simulink model "F1WingAeroDemo"  (R2025b)
settings: Solver=ode45  StartTime=0.0  StopTime=20  RelTol=1e-3
settings Model: Creator=logan78  LastModifiedBy=logan78

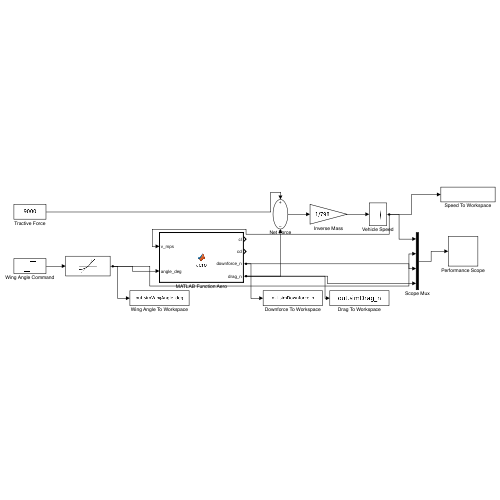
[thumbnail: Simulink's stored preview of the top-level diagram]
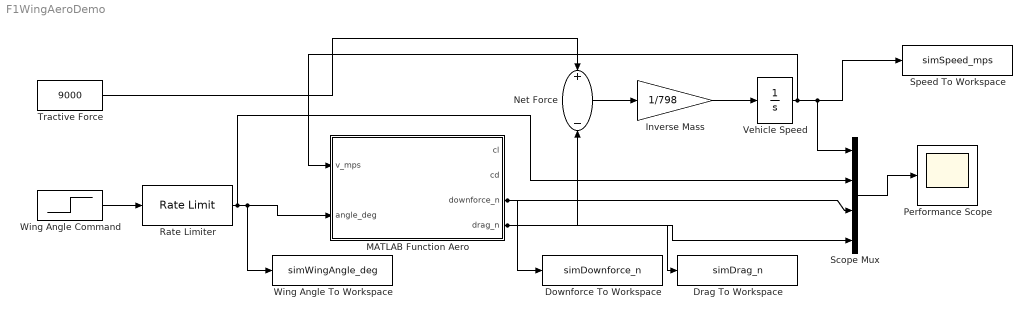
== system F1WingAeroDemo ==
  Downforce To Workspace : ToWorkspace  VariableName=simDownforce_n  SaveFormat=Structure With Time  SampleTime=-1
  Drag To Workspace : ToWorkspace  VariableName=simDrag_n  SaveFormat=Structure With Time  SampleTime=-1
  Inverse Mass : Gain  Gain=1/798
  MATLAB Function Aero : MATLAB Function  TreatAsAtomicUnit=on
  Net Force : Sum  Inputs=+-
  Performance Scope : Scope
  Rate Limiter : RateLimiter  RisingSlewLimit=90  FallingSlewLimit=-90  SampleTimeMode=inherited
  Scope Mux : Mux
  Speed To Workspace : ToWorkspace  VariableName=simSpeed_mps  SaveFormat=Structure With Time  SampleTime=-1
  Tractive Force : Constant  Value=9000
  Vehicle Speed : Integrator  InitialCondition=20  LimitOutput=on  LowerSaturationLimit=0
  Wing Angle Command : Step  Time=5  Before=5  After=18  SampleTime=0
  Wing Angle To Workspace : ToWorkspace  VariableName=simWingAngle_deg  SaveFormat=Structure With Time  SampleTime=-1
  wires:
  Tractive Force/1 -> Net Force/1
  Net Force/1 -> Inverse Mass/1
  Inverse Mass/1 -> Vehicle Speed/1
  Vehicle Speed/1 -> Scope Mux/1, Speed To Workspace/1, MATLAB Function Aero/1(v_mps)
  Wing Angle Command/1 -> Rate Limiter/1
  Rate Limiter/1 -> MATLAB Function Aero/2(angle_deg), Wing Angle To Workspace/1, Scope Mux/2
  MATLAB Function Aero/3(downforce_n) -> Scope Mux/3, Downforce To Workspace/1
  MATLAB Function Aero/4(drag_n) -> Net Force/2, Scope Mux/4, Drag To Workspace/1
  Scope Mux/1 -> Performance Scope/1

== matlab function F1WingAeroDemo/MATLAB Function Aero ==
  data: v_mps input; cl output; angle_deg input; cd output; downforce_n output; drag_n output
function [cl,cd,downforce_n,drag_n] = aero(v_mps,angle_deg)
% Representative educational model; SI units.
rho=1.225; A=1.5; Aw=0.72; AR=1.0^2/Aw; e=0.78; a0=6.1;
a=a0/(1+a0/(pi*e*AR)); stall=18; width=7;
clw=a*deg2rad(min(angle_deg,stall)+2);
if angle_deg>stall, clw=a*deg2rad(stall+2)*exp(-(angle_deg-stall)/width); end
cdw=0.055+clw^2/(pi*e*AR)+0.55*(1-exp(-(max(angle_deg-stall,0)/width)^2));
cl=2.4+clw*Aw/A; cd=0.78+cdw*Aw/A; q=0.5*rho*max(v_mps,0)^2;
downforce_n=q*A*cl; drag_n=q*A*cd;
end
